simulink model "controller_Harness"  (R2023b)
settings: Solver=VariableStepAuto  StartTime=0.0  StopTime=40  FixedStep=1/100  RelTol=1e-3
libraries: simulink x4
settings Model: Creator=Matteo  LastModifiedBy=Matteo
settings OptimizationCC: ReuseModelBlockBuffer=off
settings DebuggingCC: UnconnectedInputMsg=warning  UnconnectedOutputMsg=warning  UnconnectedLineMsg=warning
settings ModelReferenceCC: EnableRefExpFcnMdlSchedulingChecks=on
settings RTWCC: DLArmComputeVersion=19.05
settings ConfigComp: CovEnable=on  CovScope=ReferencedModels  CovIncludeTopModel=off  CovMetricSettings=dcwe  CovModelRefEnable=on

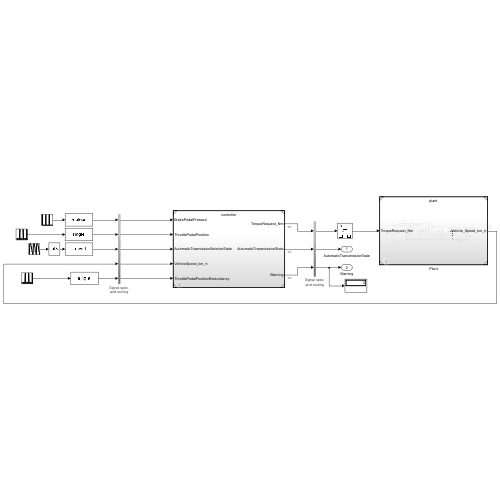
[thumbnail: Simulink's stored preview of the top-level diagram]
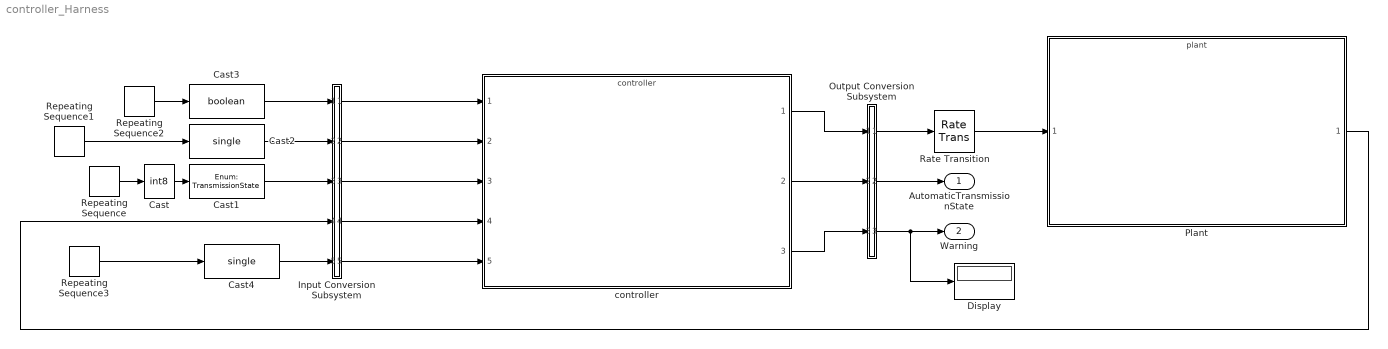
== system controller_Harness ==
  Cast : DataTypeConversion  OutDataTypeStr=int8  SaturateOnIntegerOverflow=off  RndMeth=Floor
  Cast1 : DataTypeConversion  OutDataTypeStr=Enum: TransmissionState  SaturateOnIntegerOverflow=off  RndMeth=Floor
  Cast2 : DataTypeConversion  OutDataTypeStr=single  SaturateOnIntegerOverflow=off  RndMeth=Floor
  Cast3 : DataTypeConversion  OutDataTypeStr=boolean  SaturateOnIntegerOverflow=off  RndMeth=Floor
  Cast4 : DataTypeConversion  OutDataTypeStr=single  SaturateOnIntegerOverflow=off  RndMeth=Floor
  Display : Display
  Input Conversion Subsystem : Subsystem  Tag=__SLT_ICS__  Description=|
      | Signal spec.
      | and routing
      settings: AttributesFormatString=%<Description>
  Output Conversion Subsystem : Subsystem  Tag=__SLT_OCS__  Description=|
      | Signal spec.
      | and routing
      settings: AttributesFormatString=%<Description>
  Plant : ModelReference  ModelNameDialog=plant  SimulationMode=Normal  ModelReferenceVersion=3.19
  Rate Transition : RateTransition
  Repeating Sequence : simulink/Sources/Repeating Sequence  rep_seq_t=[0 4 17 18 24 25 27.5 28 36 37 40]  rep_seq_y=[0 4 4 3 3 2 2 1 1 0 0]
  Repeating Sequence1 : simulink/Sources/Repeating Sequence  rep_seq_t=[0 4 6 7 8 12 13 14 17 18 20 22 23 24 25 26 27 28 30 35 36 37 38 39 40]  rep_seq_y=[0 0 1 1.1 1 0.2 0.01 0.01 0 0 1 0 -0.1 0 0 0 0.05 -0.05 0 1.2 10 0 0.3 -0.3 0]
  Repeating Sequence2 : simulink/Sources/Repeating Sequence  rep_seq_t=[0 0.1 3 3.01 40]  rep_seq_y=[0 1 1 0 0]
  Repeating Sequence3 : simulink/Sources/Repeating Sequence  rep_seq_t=[0 4 6 7 8 12 13 14 17 18 20 22 23 24 25 26 27 28 30 35 36 37 38 39 40]  rep_seq_y=[0 0 1 1.1 1 0.34 0.01 0.01 0 0 1 0 -0.3 0 0 0 0.05 -0.05 0 1.2 10 0 0.3 -0.3 0]
  controller : ModelReference  ModelNameDialog=controller  SimulationMode=Normal  ModelReferenceVersion=5.108
  AutomaticTransmissionState : Outport
  Warning : Outport  Port=2
  wires:
  Cast3/1 -> Input Conversion Subsystem/1(Inport_1)
  Cast1/1 -> Input Conversion Subsystem/3(Inport_3)
  Plant/1 -> Input Conversion Subsystem/4(Inport_4)
  Cast2/1 -> Input Conversion Subsystem/2(Inport_2)
  Output Conversion Subsystem/1(Outport_1) -> Rate Transition/1
  Output Conversion Subsystem/2(Outport_2) -> AutomaticTransmissionState/1
  Output Conversion Subsystem/3(Outport_3) -> Display/1, Warning/1
  Input Conversion Subsystem/1(Outport_1) -> controller/1
  Input Conversion Subsystem/2(Outport_2) -> controller/2
  Input Conversion Subsystem/3(Outport_3) -> controller/3
  Input Conversion Subsystem/4(Outport_4) -> controller/4
  Input Conversion Subsystem/5(Outport_5) -> controller/5
  controller/1 -> Output Conversion Subsystem/1(Inport_1)
  controller/2 -> Output Conversion Subsystem/2(Inport_2)
  controller/3 -> Output Conversion Subsystem/3(Inport_3)
  Repeating Sequence/1 -> Cast/1
  Cast/1 -> Cast1/1
  Repeating Sequence1/1 -> Cast2/1
  Repeating Sequence2/1 -> Cast3/1
  Rate Transition/1 -> Plant/1
  Repeating Sequence3/1 -> Cast4/1
  Cast4/1 -> Input Conversion Subsystem/5(Inport_5)

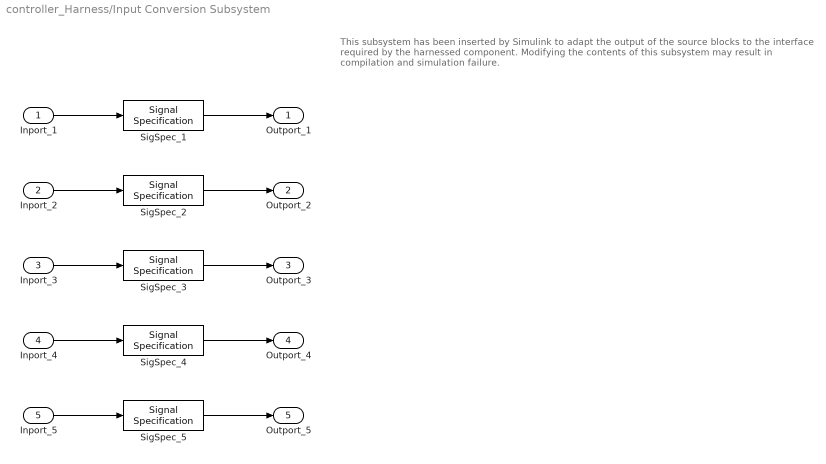
== system controller_Harness/Input Conversion Subsystem ==
  note: This subsystem has been inserted by Simulink to adapt the output of the source blocks to the interface required by the harnessed component.
      |  Modifying the contents of this subsystem may result in compilation and simulation failure.
  Inport_1 : Inport
  Inport_2 : Inport  Port=2
  Inport_3 : Inport  Port=3
  Inport_4 : Inport  Port=4
  Inport_5 : Inport  Port=5
  SigSpec_1 : SignalSpecification  OutDataTypeStr=boolean  Dimensions=[1]  SampleTime=0.01
  SigSpec_2 : SignalSpecification  OutDataTypeStr=single  Dimensions=[1]  SampleTime=0.01
  SigSpec_3 : SignalSpecification  OutDataTypeStr=Enum: TransmissionState  Dimensions=[1]  SampleTime=0.01
  SigSpec_4 : SignalSpecification  OutDataTypeStr=single  Unit=km/h  Dimensions=[1]  SampleTime=0.01
  SigSpec_5 : SignalSpecification  OutDataTypeStr=single  Dimensions=[1]  SampleTime=0.01
  Outport_1 : Outport
  Outport_2 : Outport  Port=2
  Outport_3 : Outport  Port=3
  Outport_4 : Outport  Port=4
  Outport_5 : Outport  Port=5
  wires:
  SigSpec_1/1 -> Outport_1/1
  Inport_1/1 -> SigSpec_1/1
  SigSpec_2/1 -> Outport_2/1
  Inport_2/1 -> SigSpec_2/1
  SigSpec_3/1 -> Outport_3/1
  Inport_3/1 -> SigSpec_3/1
  SigSpec_4/1 -> Outport_4/1
  Inport_4/1 -> SigSpec_4/1
  SigSpec_5/1 -> Outport_5/1
  Inport_5/1 -> SigSpec_5/1

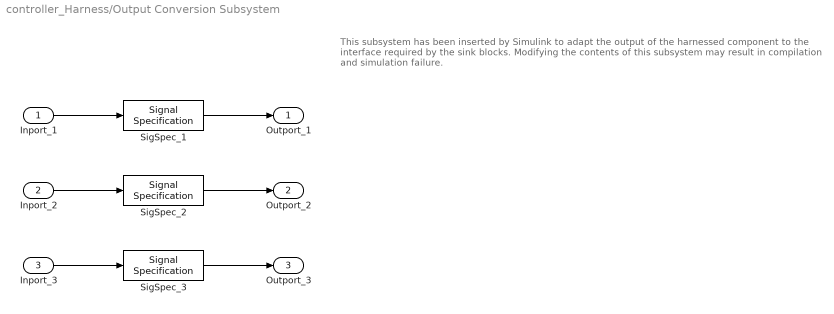
== system controller_Harness/Output Conversion Subsystem ==
  note: This subsystem has been inserted by Simulink to adapt the output of the harnessed component to the interface required by the sink blocks.
      |  Modifying the contents of this subsystem may result in compilation and simulation failure.
  Inport_1 : Inport
  Inport_2 : Inport  Port=2
  Inport_3 : Inport  Port=3
  SigSpec_1 : SignalSpecification  OutDataTypeStr=single  Unit=N*m  Dimensions=[1]  SampleTime=0.01
  SigSpec_2 : SignalSpecification  OutDataTypeStr=Enum: TransmissionState  Dimensions=[1]  SampleTime=0.01
  SigSpec_3 : SignalSpecification  OutDataTypeStr=boolean  Dimensions=[1]  SampleTime=0.01
  Outport_1 : Outport
  Outport_2 : Outport  Port=2
  Outport_3 : Outport  Port=3
  wires:
  Inport_1/1 -> SigSpec_1/1
  SigSpec_1/1 -> Outport_1/1
  Inport_2/1 -> SigSpec_2/1
  SigSpec_2/1 -> Outport_2/1
  Inport_3/1 -> SigSpec_3/1
  SigSpec_3/1 -> Outport_3/1
